simulink model "IMC"  (R2023b)
settings: Solver=VariableStepAuto  StartTime=0.0  StopTime=400  RelTol=1e-3
settings Model: Creator=86189  LastModifiedBy=86189

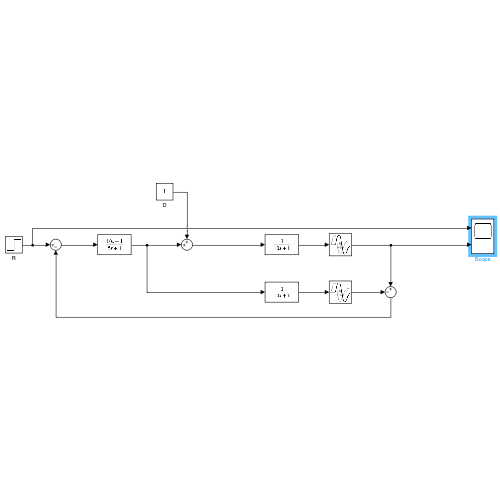
[thumbnail: Simulink's stored preview of the top-level diagram]
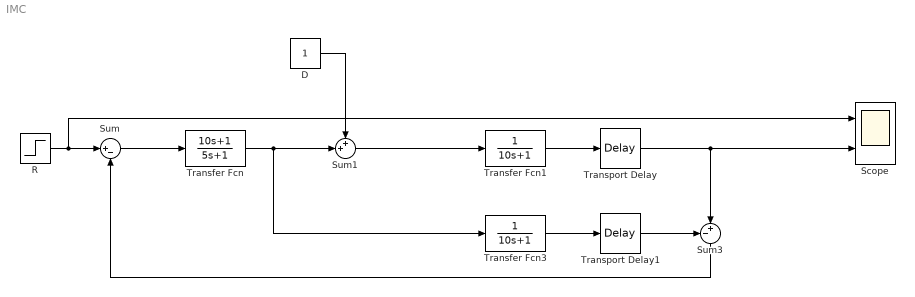
== system IMC ==
  D : Constant
  R : Step  SampleTime=0
  Scope : Scope  NumInputPorts=2
  Sum : Sum  Inputs=|+-
  Sum1 : Sum  Inputs=++|
  Sum3 : Sum  Inputs=-+|
  Transfer Fcn : TransferFcn  Numerator=[10 1]  Denominator=[5 1]
  Transfer Fcn1 : TransferFcn  Denominator=[10 1]
  Transfer Fcn3 : TransferFcn  Denominator=[10 1]
  Transport Delay : TransportDelay  DelayTime=10
  Transport Delay1 : TransportDelay  DelayTime=8
  wires:
  Sum/1 -> Transfer Fcn/1
  Transfer Fcn/1 -> Sum1/2, Transfer Fcn3/1
  Sum1/1 -> Transfer Fcn1/1
  Transfer Fcn1/1 -> Transport Delay/1
  Transport Delay/1 -> Sum3/2, Scope/2
  Transfer Fcn3/1 -> Transport Delay1/1
  Sum3/1 -> Sum/2
  R/1 -> Scope/1, Sum/1
  D/1 -> Sum1/1
  Transport Delay1/1 -> Sum3/1
